simulink model "WP_SIM"  (R2023b)
settings: Solver=ode3  StartTime=0.0  StopTime=262080  FixedStep=5.0  RelTol=1e-3
values from neighbouring files (symbols this model uses):
  a = 6    [WP_SRC.m]
  b = 0.1    [WP_SRC.m]
  C = 3e6    (= 3000000)    [WP_SRC.m]
  Q_wp_max = 5000    [WP_SRC.m]
  R = 3    [WP_SRC.m]
settings Model: Creator=johan  LastModifiedBy=johan

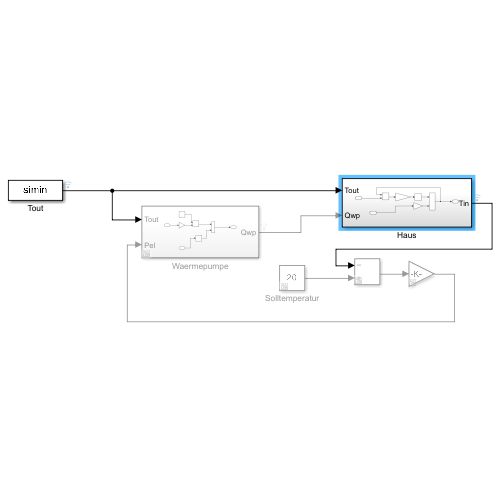
[thumbnail: Simulink's stored preview of the top-level diagram]
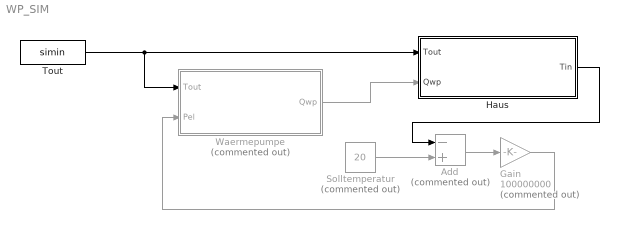
== system WP_SIM ==
  Add : Sum  Commented=on  Inputs=-+
  Gain : Gain  Commented=on  Gain=100000000
  Haus : Subsystem
  Solltemperatur : Constant  Commented=on  Value=20
  Tout : FromWorkspace  VariableName=simin  OutputAfterFinalValue=Holding final value
  Waermepumpe : Subsystem  Commented=on
  wires:
  Waermepumpe/1(Qwp) -> Haus/2(Qwp)
  Tout/1 -> Haus/1(Tout), Waermepumpe/1(Tout)
  Haus/1(Tin) -> Add/1
  Solltemperatur/1 -> Add/2
  Add/1 -> Gain/1
  Gain/1 -> Waermepumpe/2(Pel)

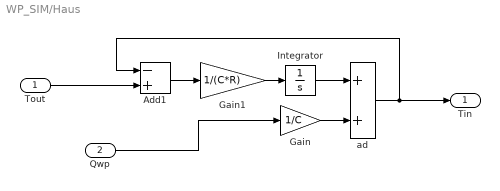
== system WP_SIM/Haus ==
  Tout : Inport
  Qwp : Inport  Port=2
  Add1 : Sum  Inputs=-+
  Gain : Gain  Gain=1/C
  Gain1 : Gain  Gain=1/(C*R)
  Integrator : Integrator  InitialCondition=20
  ad : Sum
  Tin : Outport
  wires:
  Gain1/1 -> Integrator/1
  Gain/1 -> ad/2
  Tout/1 -> Add1/2
  Integrator/1 -> ad/1
  ad/1 -> Tin/1, Add1/1
  Add1/1 -> Gain1/1
  Qwp/1 -> Gain/1

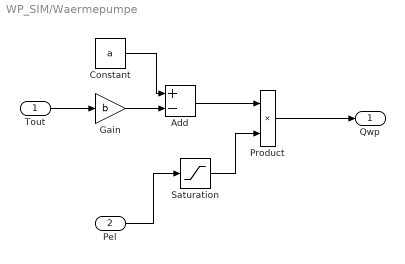
== system WP_SIM/Waermepumpe ==
  Tout : Inport
  Pel : Inport  Port=2
  Add : Sum  Inputs=+-
  Constant : Constant  Value=a
  Gain : Gain  Gain=b
  Product : Product
  Saturation : Saturate  UpperLimit=Q_wp_max  LowerLimit=0
  Qwp : Outport
  wires:
  Add/1 -> Product/1
  Gain/1 -> Add/2
  Constant/1 -> Add/1
  Product/1 -> Qwp/1
  Tout/1 -> Gain/1
  Saturation/1 -> Product/2
  Pel/1 -> Saturation/1
